simulink model "Evita_paredes"  (R2023b)
settings: Solver=FixedStepAuto  StartTime=0.0  StopTime=inf  RelTol=1e-3  EnableMultiTasking=on
settings Model: ExtModeTrigDuration=2  Creator=Manuel  LastModifiedBy=Manuel
settings SolverCC: AutoInsertRateTranBlk=on
settings OptimizationCC: EnhancedBackFolding=on  PassReuseOutputArgsAs=Individual arguments  ZeroExternalMemoryAtStartup=off  ZeroInternalMemoryAtStartup=off  MaxStackSize=64  OptimizeBlockOrder=speed  DifferentSizesBufferReuse=on  OptimizationCustomize=off  EfficientTunableParamExpr=on
settings DebuggingCC: ParameterTunabilityLossMsg=error
settings HardwareCC: ProdBitPerInt=16  ProdBitPerPointer=16  ProdBitPerSizeT=16  ProdBitPerPtrDiffT=16  ProdLargestAtomicFloat=None  ProdWordSize=8  ProdHWDeviceType=Atmel->AVR
settings SFSimCC: MATLABDynamicMemAlloc=off
settings RTWCC: Description=Embedded Coder  SystemTargetFile=ert.tlc  HardwareBoard=Arduino Mega 2560  TemplateMakefile=ert_default_tmf  Toolchain=Arduino AVR  BuildConfiguration=Faster Runs
settings CodeAppCC: ForceParamTrailComments=on  IgnoreCustomStorageClasses=off  OperatorAnnotations=on  SimulinkDataObjDesc=on  SFDataObjDesc=on  InsertBlockDesc=on
settings ERTTargetCC: SupportContinuousTime=on  SupportVariableSizeSignals=on  ExtModeTransport=3  ExtModeStaticAlloc=on  ExtModeAutomaticAllocSize=off  ExtModeStaticAllocSize=2048  ExtModeMexFile=ext_xcp  ExtModeIntrfLevel=Level2 - Open

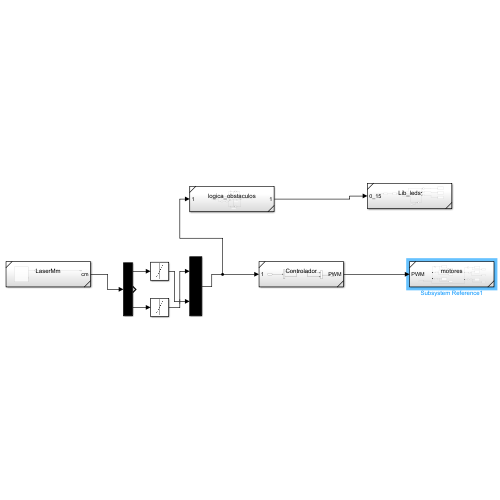
[thumbnail: Simulink's stored preview of the top-level diagram]
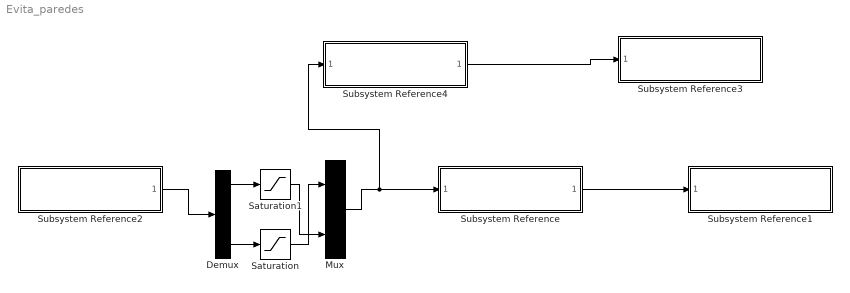
== system Evita_paredes ==
  Demux : Demux  Outputs=3
  Mux : Mux  Inputs=2
  Saturation : Saturate  UpperLimit=200  LowerLimit=-250
  Saturation1 : Saturate  UpperLimit=200  LowerLimit=-250
  Subsystem Reference : Subsystem  ReferencedSubsystem=Controlador
  Subsystem Reference1 : Subsystem  ReferencedSubsystem=motores
  Subsystem Reference2 : Subsystem  ReferencedSubsystem=LaserMm
  Subsystem Reference3 : Subsystem  ReferencedSubsystem=Lib_leds
  Subsystem Reference4 : Subsystem  ReferencedSubsystem=logica_obstaculos
  wires:
  Subsystem Reference/1 -> Subsystem Reference1/1
  Mux/1 -> Subsystem Reference4/1, Subsystem Reference/1
  Subsystem Reference2/1 -> Demux/1
  Demux/3 -> Saturation/1
  Saturation/1 -> Mux/1
  Demux/1 -> Saturation1/1
  Saturation1/1 -> Mux/2
  Subsystem Reference4/1 -> Subsystem Reference3/1
